simulink library "boothParameterConversionSim_ul"  (R2020a)
settings: Solver=VariableStepAuto  StartTime=0.0  StopTime=10.0  RelTol=1e-3
settings Model: Creator=Ayaz  LastModifiedBy=Ayaz

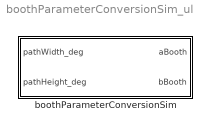
== system boothParameterConversionSim_ul ==
  boothParameterConversionSim : Subsystem

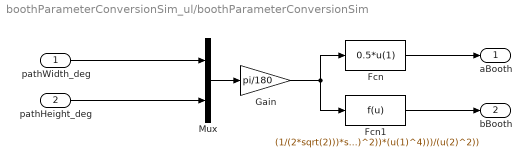
== system boothParameterConversionSim_ul/boothParameterConversionSim ==
  pathWidth_deg : Inport  PortDimensions=1
  pathHeight_deg : Inport  Port=2  PortDimensions=1
  Fcn : Fcn  Expr=0.5*u(1)
  Fcn1 : Fcn  Expr=(1/(2*sqrt(2)))*sqrt(-(u(1)^2)+sqrt(((u(2)^2)*(4+(u(2)^2))*(u(1)^4)))/(u(2)^2))
  Gain : Gain  Gain=pi/180
  Mux : Mux  Inputs=2
  aBooth : Outport  PortDimensions=1
  bBooth : Outport  Port=2  PortDimensions=1
  wires:
  Fcn/1 -> aBooth/1
  Fcn1/1 -> bBooth/1
  pathWidth_deg/1 -> Mux/1
  Gain/1 -> Fcn1/1, Fcn/1
  pathHeight_deg/1 -> Mux/2
  Mux/1 -> Gain/1
